simulink model "BaiTapDKSTDD"  (R2019a)
settings: Solver=VariableStepAuto  StartTime=0.0  StopTime=10.0  RelTol=1e-3
libraries: dspswit3 x1, powerlib x1
settings Model: Creator=Admin  LastModifiedBy=Admin

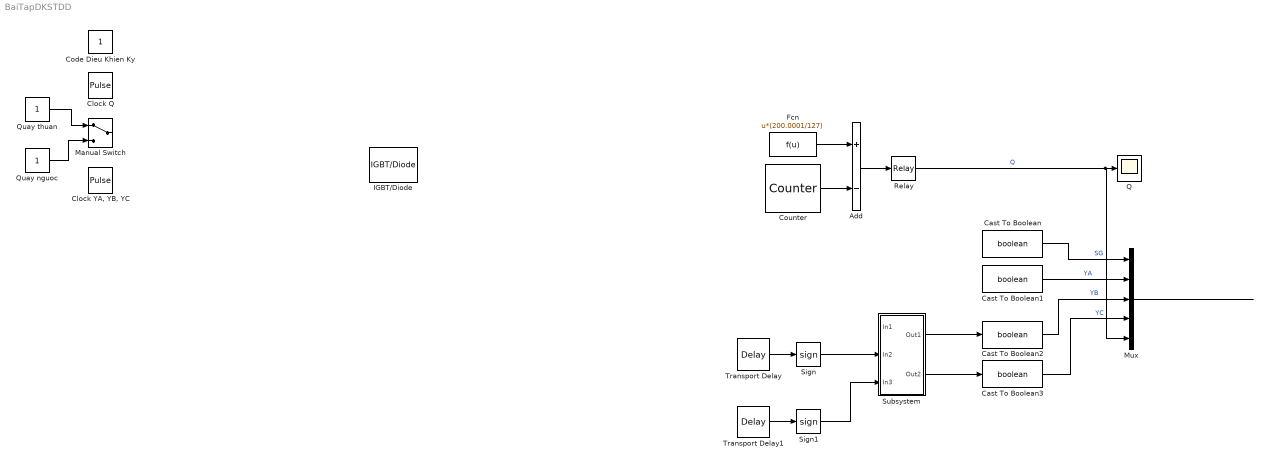
== system BaiTapDKSTDD ==
  Add : Sum  Inputs=+-
  Cast To Boolean{,1..3} (4 alike) : DataTypeConversion  OutDataTypeStr=boolean
  Clock Q : DiscretePulseGenerator  PulseType=Time based  Period=0.00000992157  PulseWidth=50
  "Clock YA, YB, YC" : DiscretePulseGenerator  PulseType=Time based  Period=0.002  PulseWidth=50
  Code Dieu Khien Ky : Constant
  Counter : dspswit3/Counter  Direction=Up  CountEvent=Rising edge  CounterSize=User defined  MaxCount=200  InitialCount=0  Output=Count  HitValue=32  ResetInput=off  SamplesPerFrame=1  Ts=1  CntDtype=double  HitDtype=Logical
  Fcn : Fcn  Expr=u*(200.0001/127)
  IGBT/Diode : powerlib/Power Electronics/IGBT//Diode  Ron=1e-3  Rs=1e5  Cs=inf  Measurements=on
      settings: SourceProductName=Simscape Electrical
  Manual Switch : ManualSwitch
  Mux : Mux  Inputs=5
  Q : Scope
  Quay nguoc : Constant
  Quay thuan : Constant
  Relay : Relay
  Sign : Signum
  Sign1 : Signum
  Subsystem : Subsystem
  Transport Delay : TransportDelay  DelayTime=0.04/3  TransDelayFeedthrough=on
  Transport Delay1 : TransportDelay  DelayTime=0.04/3  TransDelayFeedthrough=on
  wires:
  Quay nguoc/1 -> Manual Switch/2
  Quay thuan/1 -> Manual Switch/1
  Transport Delay/1 -> Sign/1
  Fcn/1 -> Add/1
  Counter/1 -> Add/2
  Add/1 -> Relay/1
  ? -> Subsystem/1(In1), Cast To Boolean/1
  ? -> Transport Delay1/1, Transport Delay/1, Cast To Boolean1/1
  Sign/1 -> Subsystem/2(In2)
  Sign1/1 -> Subsystem/3(In3)
  Subsystem/1(Out1) -> Cast To Boolean2/1
  Subsystem/2(Out2) -> Cast To Boolean3/1
  Relay/1 -> Mux/5, Q/1  "Q"
  Cast To Boolean/1 -> Mux/1  "SG"
  Cast To Boolean1/1 -> Mux/2  "YA"
  Cast To Boolean2/1 -> Mux/3  "YB"
  Cast To Boolean3/1 -> Mux/4  "YC"
  Mux/1 -> ?
  Transport Delay1/1 -> Sign1/1

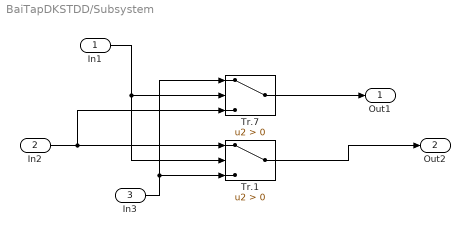
== system BaiTapDKSTDD/Subsystem ==
  In1 : Inport
  In2 : Inport  Port=2
  In3 : Inport  Port=3
  Tr.1 : Switch  Criteria=u2 > Threshold
  Tr.7 : Switch  Criteria=u2 > Threshold
  Out1 : Outport
  Out2 : Outport  Port=2
  wires:
  Tr.1/1 -> Out2/1
  In1/1 -> Tr.1/2, Tr.7/2
  In2/1 -> Tr.7/3, Tr.1/1
  In3/1 -> Tr.1/3, Tr.7/1
  Tr.7/1 -> Out1/1
